simulink model "ctrl_TT"  (R2022b)
settings: Solver=FixedStepAuto  StartTime=0.0  StopTime=Tf  FixedStep=0.05  RelTol=1e-3
InitFcn:
  | run;
StopFcn:
  | save('testdata')
undefined symbols (not defined in the file): Ba_0, Bb, Bv_0, Bx_0, Cp, Cp_prime, d, dA_BP1, dA_BP2, dA_Hull, dA_PH, dA_Sail, dA_SProot, dA_X1a, dA_X1b, dA_X2a, dA_X2b, dA_X3a, dA_X3b, dA_X4a, dA_X4b, Ixx, Ixy, Ixz, Iyy, Iyz, Izz, Mb, n_BP1, n_BP2, n_Hull, n_PH, n_Sail, n_SProot, n_X2a, n_X2b, n_X3a, n_X4a, n_X4b, nt_BP1, nt_BP2, nt_Hull, nt_PH, nt_Sail, nt_SProot, nt_X1a, nt_X1b, nt_X2a, nt_X2b, nt_X3a, nt_X3b, nt_X4a, nt_X4b, Seastate, Tf, vt1_BP1, vt1_BP2, vt1_Hull, vt1_PH, vt1_Sail ... (+44)
libraries: simulink x8, sharedtransform x2, dspmathops x2
(part 4 of 5)

== matlab function ctrl_TT/HDM/HDM B3/Wave, Virtual Mass and Hydrostatic/Wave Particle Motions/Hydrostatic Forces and Moments/Subsystem/MATLAB Function1 ==
  data: time input; Xearth input; Fx_total output; vert1 input; vert2 input; vert3 input; dA input; ntri input; normal input; A_wave input; k_wave input; w_wave input; rho input; g input; Fy_total output; Fz_total output; Mx_total output; My_total output; Mz_total output; Zb input
function [Fx_total,Fy_total,Fz_total,Mx_total,My_total,Mz_total]= fcn(time,Xearth,vert1,vert2,vert3,dA,ntri,normal,A_wave,k_wave,w_wave,rho,g,Zb)
x_e=Xearth(1); y_e=Xearth(2); z_e=Xearth(3);
phi=Xearth(4); theta=Xearth(5); psi=Xearth(6);

RMat=[cos(theta)*cos(psi) -cos(phi)*sin(psi)+sin(phi)*sin(theta)*cos(psi)  sin(phi)*sin(psi)+cos(phi)*sin(theta)*cos(psi); ...
      cos(theta)*sin(psi)  cos(phi)*cos(psi)+sin(phi)*sin(theta)*sin(psi) -sin(phi)*cos(psi)+cos(phi)*sin(theta)*sin(psi); ...
     -sin(theta)                             sin(phi)*cos(theta)                             cos(phi)*cos(theta)];  

%position of mid points in earth coordinate;
mp1=zeros(ntri,3);
mp2=zeros(ntri,3);
mp3=zeros(ntri,3);
nA =zeros(ntri,3);

P1=zeros(ntri,1);
P2=zeros(ntri,1);
P3=zeros(ntri,1);

%position vector of mid points from the CG
r1=zeros(ntri,3);
r2=zeros(ntri,3);
r3=zeros(ntri,3);
v1_w=zeros(ntri,3);
v2_w=zeros(ntri,3);
v3_w=zeros(ntri,3);
n_w=zeros(ntri,3);

%Area of triangle, product of area and unit normal, position vector to each mid-point
for i=1:ntri
    %Area of each triangle
    A=[vert2(i,1)-vert1(i,1); vert2(i,2)-vert1(i,2); vert2(i,3)-vert1(i,3);];
    B=[vert3(i,1)-vert1(i,1); vert3(i,2)-vert1(i,2); vert3(i,3)-vert1(i,3);];
    C=[normal(i,1); normal(i,2); normal(i,3);];
        
    %A*n vector calculation
    for j=1:3
        nA(i,j)=dA(i).*C(j);    
    end
    
    %position vector to each mid point of each edge
    for j=1:3
        r1(i,j)=0.5*(vert1(i,j)+vert2(i,j));
        r2(i,j)=0.5*(vert1(i,j)+vert3(i,j));
        r3(i,j)=0.5*(vert2(i,j)+vert3(i,j));
    end
end

%computing mid point location between vertices in earth coordinate
for i=1:ntri
    MP1=RMat*[r1(i,1); r1(i,2); r1(i,3);]+[x_e; y_e; z_e;];
    MP2=RMat*[r2(i,1); r2(i,2); r2(i,3);]+[x_e; y_e; z_e;];
    MP3=RMat*[r3(i,1); r3(i,2); r3(i,3);]+[x_e; y_e; z_e;];
    
    v1i=RMat*[vert1(i,1); vert1(i,2); vert1(i,3);]+[x_e; y_e; z_e;];
    v2i=RMat*[vert2(i,1); vert2(i,2); vert2(i,3);]+[x_e; y_e; z_e;];
    v3i=RMat*[vert3(i,1); vert3(i,2); vert3(i,3);]+[x_e; y_e; z_e;];
   
    for j=1:3
        v1_w(i,j)=v1i(j); v2_w(i,j)=v2i(j); v3_w(i,j)=v3i(j); 
        mp1(i,j)=MP1(j);  mp2(i,j)=MP2(j);  mp3(i,j)=MP3(j);
    end
end

for i=1:ntri
    A=[v2_w(i,1)-v1_w(i,1); v2_w(i,2)-v1_w(i,2); v2_w(i,3)-v1_w(i,3);];
    B=[v3_w(i,1)-v1_w(i,1); v3_w(i,2)-v1_w(i,2); v3_w(i,3)-v1_w(i,3);];
    n=cross(A,B)/norm(cross(A,B));
    dA(i,1)=0.5*norm(cross(A,B));
    n_w(i,1)=n(1); n_w(i,2)=n(2); n_w(i,3)=n(3);
end


%computing forces and moments for each triangle
Fx_total=0; Fy_total=0; Fz_total=0;
Mx_total=0; My_total=0; Mz_total=0;

for i=1:ntri
    p1=-rho*g*(mp1(i,3)-A_wave*exp(k_wave.*mp1(i,3)).*sin(k_wave*mp1(i,1)-w_wave.*time));
    p2=-rho*g*(mp2(i,3)-A_wave*exp(k_wave.*mp2(i,3)).*sin(k_wave*mp2(i,1)-w_wave.*time));
    p3=-rho*g*(mp3(i,3)-A_wave*exp(k_wave.*mp3(i,3)).*sin(k_wave*mp3(i,1)-w_wave.*time));
    
    dFx=-nA(i,1)*(p1+p2+p3)./3;
    dFy=-nA(i,2)*(p1+p2+p3)./3;
    dFz=-nA(i,3)*(p1+p2+p3)./3;
    
    dP =-p1.*[r1(i,1); r1(i,2); r1(i,3)-Zb;]...
        -p2.*[r2(i,1); r2(i,2); r2(i,3)-Zb;]...
        -p3.*[r3(i,1); r3(i,2); r3(i,3)-Zb;];
    N =[nA(i,1); nA(i,2); nA(i,3);];
    dM=cross(dP,N);
    Fx_total=Fx_total+dFx;
    Fy_total=Fy_total+dFy;
    Fz_total=Fz_total+dFz;
    Mx_total=Mx_total+dM(1)/3;
    My_total=My_total+dM(2)/3;
    Mz_total=Mz_total+dM(3)/3;
end
end

== matlab function ctrl_TT/HDM/HDM B3/Wave, Virtual Mass and Hydrostatic/Wave Particle Motions/Hydrostatic Forces and Moments/Subsystem/MATLAB Function3 ==
  data: time input; Xearth input; Fx_total output; vert1 input; vert2 input; vert3 input; dA input; ntri input; normal input; A_wave input; k_wave input; w_wave input; rho input; g input; Fy_total output; Fz_total output; Mx_total output; My_total output; Mz_total output; Zb input
function [Fx_total,Fy_total,Fz_total,Mx_total,My_total,Mz_total]= fcn(time,Xearth,vert1,vert2,vert3,dA,ntri,normal,A_wave,k_wave,w_wave,rho,g,Zb)
x_e=Xearth(1); y_e=Xearth(2); z_e=Xearth(3);
phi=Xearth(4); theta=Xearth(5); psi=Xearth(6);

RMat=[cos(theta)*cos(psi) -cos(phi)*sin(psi)+sin(phi)*sin(theta)*cos(psi)  sin(phi)*sin(psi)+cos(phi)*sin(theta)*cos(psi); ...
      cos(theta)*sin(psi)  cos(phi)*cos(psi)+sin(phi)*sin(theta)*sin(psi) -sin(phi)*cos(psi)+cos(phi)*sin(theta)*sin(psi); ...
     -sin(theta)                             sin(phi)*cos(theta)                             cos(phi)*cos(theta)];  

%position of mid points in earth coordinate;
mp1=zeros(ntri,3);
mp2=zeros(ntri,3);
mp3=zeros(ntri,3);
nA =zeros(ntri,3);

P1=zeros(ntri,1);
P2=zeros(ntri,1);
P3=zeros(ntri,1);

%position vector of mid points from the CG
r1=zeros(ntri,3);
r2=zeros(ntri,3);
r3=zeros(ntri,3);
v1_w=zeros(ntri,3);
v2_w=zeros(ntri,3);
v3_w=zeros(ntri,3);
n_w=zeros(ntri,3);

%Area of triangle, product of area and unit normal, position vector to each mid-point
for i=1:ntri
    %Area of each triangle
    A=[vert2(i,1)-vert1(i,1); vert2(i,2)-vert1(i,2); vert2(i,3)-vert1(i,3);];
    B=[vert3(i,1)-vert1(i,1); vert3(i,2)-vert1(i,2); vert3(i,3)-vert1(i,3);];
    C=[normal(i,1); normal(i,2); normal(i,3);];
        
    %A*n vector calculation
    for j=1:3
        nA(i,j)=dA(i).*C(j);    
    end
    
    %position vector to each mid point of each edge
    for j=1:3
        r1(i,j)=0.5*(vert1(i,j)+vert2(i,j));
        r2(i,j)=0.5*(vert1(i,j)+vert3(i,j));
        r3(i,j)=0.5*(vert2(i,j)+vert3(i,j));
    end
end

%computing mid point location between vertices in earth coordinate
for i=1:ntri
    MP1=RMat*[r1(i,1); r1(i,2); r1(i,3);]+[x_e; y_e; z_e;];
    MP2=RMat*[r2(i,1); r2(i,2); r2(i,3);]+[x_e; y_e; z_e;];
    MP3=RMat*[r3(i,1); r3(i,2); r3(i,3);]+[x_e; y_e; z_e;];
    
    v1i=RMat*[vert1(i,1); vert1(i,2); vert1(i,3);]+[x_e; y_e; z_e;];
    v2i=RMat*[vert2(i,1); vert2(i,2); vert2(i,3);]+[x_e; y_e; z_e;];
    v3i=RMat*[vert3(i,1); vert3(i,2); vert3(i,3);]+[x_e; y_e; z_e;];
   
    for j=1:3
        v1_w(i,j)=v1i(j); v2_w(i,j)=v2i(j); v3_w(i,j)=v3i(j); 
        mp1(i,j)=MP1(j);  mp2(i,j)=MP2(j);  mp3(i,j)=MP3(j);
    end
end

for i=1:ntri
    A=[v2_w(i,1)-v1_w(i,1); v2_w(i,2)-v1_w(i,2); v2_w(i,3)-v1_w(i,3);];
    B=[v3_w(i,1)-v1_w(i,1); v3_w(i,2)-v1_w(i,2); v3_w(i,3)-v1_w(i,3);];
    n=cross(A,B)/norm(cross(A,B));
    dA(i,1)=0.5*norm(cross(A,B));
    n_w(i,1)=n(1); n_w(i,2)=n(2); n_w(i,3)=n(3);
end



%computing forces and moments for each triangle
Fx_total=0; Fy_total=0; Fz_total=0;
Mx_total=0; My_total=0; Mz_total=0;

for i=1:ntri
    p1=-rho*g*(mp1(i,3)-A_wave*exp(k_wave.*mp1(i,3)).*sin(k_wave*mp1(i,1)-w_wave.*time));
    p2=-rho*g*(mp2(i,3)-A_wave*exp(k_wave.*mp2(i,3)).*sin(k_wave*mp2(i,1)-w_wave.*time));
    p3=-rho*g*(mp3(i,3)-A_wave*exp(k_wave.*mp3(i,3)).*sin(k_wave*mp3(i,1)-w_wave.*time));
    
    dFx=-nA(i,1)*(p1+p2+p3)./3;
    dFy=-nA(i,2)*(p1+p2+p3)./3;
    dFz=-nA(i,3)*(p1+p2+p3)./3;
    
    dP =-p1.*[r1(i,1); r1(i,2); r1(i,3)-Zb;]...
        -p2.*[r2(i,1); r2(i,2); r2(i,3)-Zb;]...
        -p3.*[r3(i,1); r3(i,2); r3(i,3)-Zb;];
    N =[nA(i,1); nA(i,2); nA(i,3);];
    dM=cross(dP,N);
    Fx_total=Fx_total+dFx;
    Fy_total=Fy_total+dFy;
    Fz_total=Fz_total+dFz;
    Mx_total=Mx_total+dM(1)/3;
    My_total=My_total+dM(2)/3;
    Mz_total=Mz_total+dM(3)/3;
end
end

== matlab function ctrl_TT/HDM/HDM B3/Wave, Virtual Mass and Hydrostatic/Wave Particle Motions/Hydrostatic Forces and Moments/Subsystem/MATLAB Function4 ==
  data: time input; Xearth input; Fx_total output; vert1 input; vert2 input; vert3 input; dA input; ntri input; normal input; A_wave input; k_wave input; w_wave input; rho input; g input; Fy_total output; Fz_total output; Mx_total output; My_total output; Mz_total output; Zb input
function [Fx_total,Fy_total,Fz_total,Mx_total,My_total,Mz_total]= fcn(time,Xearth,vert1,vert2,vert3,dA,ntri,normal,A_wave,k_wave,w_wave,rho,g,Zb)
x_e=Xearth(1); y_e=Xearth(2); z_e=Xearth(3);
phi=Xearth(4); theta=Xearth(5); psi=Xearth(6);

RMat=[cos(theta)*cos(psi) -cos(phi)*sin(psi)+sin(phi)*sin(theta)*cos(psi)  sin(phi)*sin(psi)+cos(phi)*sin(theta)*cos(psi); ...
      cos(theta)*sin(psi)  cos(phi)*cos(psi)+sin(phi)*sin(theta)*sin(psi) -sin(phi)*cos(psi)+cos(phi)*sin(theta)*sin(psi); ...
     -sin(theta)                             sin(phi)*cos(theta)                             cos(phi)*cos(theta)];  

%position of mid points in earth coordinate;
mp1=zeros(ntri,3);
mp2=zeros(ntri,3);
mp3=zeros(ntri,3);
nA =zeros(ntri,3);

P1=zeros(ntri,1);
P2=zeros(ntri,1);
P3=zeros(ntri,1);

%position vector of mid points from the CG
r1=zeros(ntri,3);
r2=zeros(ntri,3);
r3=zeros(ntri,3);
v1_w=zeros(ntri,3);
v2_w=zeros(ntri,3);
v3_w=zeros(ntri,3);
n_w=zeros(ntri,3);

%Area of triangle, product of area and unit normal, position vector to each mid-point
for i=1:ntri
    %Area of each triangle
    A=[vert2(i,1)-vert1(i,1); vert2(i,2)-vert1(i,2); vert2(i,3)-vert1(i,3);];
    B=[vert3(i,1)-vert1(i,1); vert3(i,2)-vert1(i,2); vert3(i,3)-vert1(i,3);];
    C=[normal(i,1); normal(i,2); normal(i,3);];
        
    %A*n vector calculation
    for j=1:3
        nA(i,j)=dA(i).*C(j);    
    end
    
    %position vector to each mid point of each edge
    for j=1:3
        r1(i,j)=0.5*(vert1(i,j)+vert2(i,j));
        r2(i,j)=0.5*(vert1(i,j)+vert3(i,j));
        r3(i,j)=0.5*(vert2(i,j)+vert3(i,j));
    end
end

%computing mid point location between vertices in earth coordinate
for i=1:ntri
    MP1=RMat*[r1(i,1); r1(i,2); r1(i,3);]+[x_e; y_e; z_e;];
    MP2=RMat*[r2(i,1); r2(i,2); r2(i,3);]+[x_e; y_e; z_e;];
    MP3=RMat*[r3(i,1); r3(i,2); r3(i,3);]+[x_e; y_e; z_e;];
    
    v1i=RMat*[vert1(i,1); vert1(i,2); vert1(i,3);]+[x_e; y_e; z_e;];
    v2i=RMat*[vert2(i,1); vert2(i,2); vert2(i,3);]+[x_e; y_e; z_e;];
    v3i=RMat*[vert3(i,1); vert3(i,2); vert3(i,3);]+[x_e; y_e; z_e;];
   
    for j=1:3
        v1_w(i,j)=v1i(j); v2_w(i,j)=v2i(j); v3_w(i,j)=v3i(j); 
        mp1(i,j)=MP1(j);  mp2(i,j)=MP2(j);  mp3(i,j)=MP3(j);
    end
end

for i=1:ntri
    A=[v2_w(i,1)-v1_w(i,1); v2_w(i,2)-v1_w(i,2); v2_w(i,3)-v1_w(i,3);];
    B=[v3_w(i,1)-v1_w(i,1); v3_w(i,2)-v1_w(i,2); v3_w(i,3)-v1_w(i,3);];
    n=cross(A,B)/norm(cross(A,B));
    dA(i,1)=0.5*norm(cross(A,B));
    n_w(i,1)=n(1); n_w(i,2)=n(2); n_w(i,3)=n(3);
end


%computing forces and moments for each triangle
Fx_total=0; Fy_total=0; Fz_total=0;
Mx_total=0; My_total=0; Mz_total=0;

for i=1:ntri
    p1=-rho*g*(mp1(i,3)-A_wave*exp(k_wave.*mp1(i,3)).*sin(k_wave*mp1(i,1)-w_wave.*time));
    p2=-rho*g*(mp2(i,3)-A_wave*exp(k_wave.*mp2(i,3)).*sin(k_wave*mp2(i,1)-w_wave.*time));
    p3=-rho*g*(mp3(i,3)-A_wave*exp(k_wave.*mp3(i,3)).*sin(k_wave*mp3(i,1)-w_wave.*time));
    
    dFx=-nA(i,1)*(p1+p2+p3)./3;
    dFy=-nA(i,2)*(p1+p2+p3)./3;
    dFz=-nA(i,3)*(p1+p2+p3)./3;
    
    dP =-p1.*[r1(i,1); r1(i,2); r1(i,3)-Zb;]...
        -p2.*[r2(i,1); r2(i,2); r2(i,3)-Zb;]...
        -p3.*[r3(i,1); r3(i,2); r3(i,3)-Zb;];
    N =[nA(i,1); nA(i,2); nA(i,3);];
    dM=cross(dP,N);
    Fx_total=Fx_total+dFx;
    Fy_total=Fy_total+dFy;
    Fz_total=Fz_total+dFz;
    Mx_total=Mx_total+dM(1)/3;
    My_total=My_total+dM(2)/3;
    Mz_total=Mz_total+dM(3)/3;
end
end

== matlab function ctrl_TT/HDM/HDM B3/Wave, Virtual Mass and Hydrostatic/Wave Particle Motions/Hydrostatic Forces and Moments/Subsystem/MATLAB Function5 ==
  data: time input; Xearth input; Fx_total output; vert1 input; vert2 input; vert3 input; dA input; ntri input; normal input; A_wave input; k_wave input; w_wave input; rho input; g input; Fy_total output; Fz_total output; Mx_total output; My_total output; Mz_total output; Zb input
function [Fx_total,Fy_total,Fz_total,Mx_total,My_total,Mz_total]= fcn(time,Xearth,vert1,vert2,vert3,dA,ntri,normal,A_wave,k_wave,w_wave,rho,g,Zb)
x_e=Xearth(1); y_e=Xearth(2); z_e=Xearth(3);
phi=Xearth(4); theta=Xearth(5); psi=Xearth(6);

RMat=[cos(theta)*cos(psi) -cos(phi)*sin(psi)+sin(phi)*sin(theta)*cos(psi)  sin(phi)*sin(psi)+cos(phi)*sin(theta)*cos(psi); ...
      cos(theta)*sin(psi)  cos(phi)*cos(psi)+sin(phi)*sin(theta)*sin(psi) -sin(phi)*cos(psi)+cos(phi)*sin(theta)*sin(psi); ...
     -sin(theta)                             sin(phi)*cos(theta)                             cos(phi)*cos(theta)];  

%position of mid points in earth coordinate;
mp1=zeros(ntri,3);
mp2=zeros(ntri,3);
mp3=zeros(ntri,3);
nA =zeros(ntri,3);

P1=zeros(ntri,1);
P2=zeros(ntri,1);
P3=zeros(ntri,1);

%position vector of mid points from the CG
r1=zeros(ntri,3);
r2=zeros(ntri,3);
r3=zeros(ntri,3);
v1_w=zeros(ntri,3);
v2_w=zeros(ntri,3);
v3_w=zeros(ntri,3);
n_w=zeros(ntri,3);

%Area of triangle, product of area and unit normal, position vector to each mid-point
for i=1:ntri
    %Area of each triangle
    A=[vert2(i,1)-vert1(i,1); vert2(i,2)-vert1(i,2); vert2(i,3)-vert1(i,3);];
    B=[vert3(i,1)-vert1(i,1); vert3(i,2)-vert1(i,2); vert3(i,3)-vert1(i,3);];
    C=[normal(i,1); normal(i,2); normal(i,3);];
        
    %A*n vector calculation
    for j=1:3
        nA(i,j)=dA(i).*C(j);    
    end
    
    %position vector to each mid point of each edge
    for j=1:3
        r1(i,j)=0.5*(vert1(i,j)+vert2(i,j));
        r2(i,j)=0.5*(vert1(i,j)+vert3(i,j));
        r3(i,j)=0.5*(vert2(i,j)+vert3(i,j));
    end
end

%computing mid point location between vertices in earth coordinate
for i=1:ntri
    MP1=RMat*[r1(i,1); r1(i,2); r1(i,3);]+[x_e; y_e; z_e;];
    MP2=RMat*[r2(i,1); r2(i,2); r2(i,3);]+[x_e; y_e; z_e;];
    MP3=RMat*[r3(i,1); r3(i,2); r3(i,3);]+[x_e; y_e; z_e;];
    
    v1i=RMat*[vert1(i,1); vert1(i,2); vert1(i,3);]+[x_e; y_e; z_e;];
    v2i=RMat*[vert2(i,1); vert2(i,2); vert2(i,3);]+[x_e; y_e; z_e;];
    v3i=RMat*[vert3(i,1); vert3(i,2); vert3(i,3);]+[x_e; y_e; z_e;];
   
    for j=1:3
        v1_w(i,j)=v1i(j); v2_w(i,j)=v2i(j); v3_w(i,j)=v3i(j); 
        mp1(i,j)=MP1(j);  mp2(i,j)=MP2(j);  mp3(i,j)=MP3(j);
    end
end

for i=1:ntri
    A=[v2_w(i,1)-v1_w(i,1); v2_w(i,2)-v1_w(i,2); v2_w(i,3)-v1_w(i,3);];
    B=[v3_w(i,1)-v1_w(i,1); v3_w(i,2)-v1_w(i,2); v3_w(i,3)-v1_w(i,3);];
    n=cross(A,B)/norm(cross(A,B));
    dA(i,1)=0.5*norm(cross(A,B));
    n_w(i,1)=n(1); n_w(i,2)=n(2); n_w(i,3)=n(3);
end



%computing forces and moments for each triangle
Fx_total=0; Fy_total=0; Fz_total=0;
Mx_total=0; My_total=0; Mz_total=0;

for i=1:ntri
    p1=-rho*g*(mp1(i,3)-A_wave*exp(k_wave.*mp1(i,3)).*sin(k_wave*mp1(i,1)-w_wave.*time));
    p2=-rho*g*(mp2(i,3)-A_wave*exp(k_wave.*mp2(i,3)).*sin(k_wave*mp2(i,1)-w_wave.*time));
    p3=-rho*g*(mp3(i,3)-A_wave*exp(k_wave.*mp3(i,3)).*sin(k_wave*mp3(i,1)-w_wave.*time));
    
    dFx=-nA(i,1)*(p1+p2+p3)./3;
    dFy=-nA(i,2)*(p1+p2+p3)./3;
    dFz=-nA(i,3)*(p1+p2+p3)./3;
    
    dP =-p1.*[r1(i,1); r1(i,2); r1(i,3)-Zb;]...
        -p2.*[r2(i,1); r2(i,2); r2(i,3)-Zb;]...
        -p3.*[r3(i,1); r3(i,2); r3(i,3)-Zb;];
    N =[nA(i,1); nA(i,2); nA(i,3);];
    dM=cross(dP,N);
    Fx_total=Fx_total+dFx;
    Fy_total=Fy_total+dFy;
    Fz_total=Fz_total+dFz;
    Mx_total=Mx_total+dM(1)/3;
    My_total=My_total+dM(2)/3;
    Mz_total=Mz_total+dM(3)/3;
end
end

== matlab function ctrl_TT/HDM/HDM B3/Wave, Virtual Mass and Hydrostatic/Wave Particle Motions/Hydrostatic Forces and Moments/X1/MATLAB Function1 ==
  data: time input; Xearth input; Fx_total output; vert1 input; vert2 input; vert3 input; dA input; ntri input; A_wave input; k_wave input; w_wave input; rho input; g input; Fy_total output; Fz_total output; Mx_total output; My_total output; Mz_total output; Zb input; EAX input; dX input; origin input; xcg input
function [Fx_total,Fy_total,Fz_total,Mx_total,My_total,Mz_total]= fcn(time,Xearth,vert1,vert2,vert3,dA,ntri,A_wave,k_wave,w_wave,rho,g,Zb,EAX,dX,origin,xcg)
%EAX=Appendage eulater angle in local coordinate
%its=number of time steps to skip writing grid
x_e=Xearth(1); y_e=Xearth(2); z_e=Xearth(3);
phi=Xearth(4); theta=Xearth(5); psi=Xearth(6);
phiX=EAX(1); thetaX=EAX(2); psiX=EAX(3);


RMat=[cos(theta)*cos(psi) -cos(phi)*sin(psi)+sin(phi)*sin(theta)*cos(psi)  sin(phi)*sin(psi)+cos(phi)*sin(theta)*cos(psi); ...
      cos(theta)*sin(psi)  cos(phi)*cos(psi)+sin(phi)*sin(theta)*sin(psi) -sin(phi)*cos(psi)+cos(phi)*sin(theta)*sin(psi); ...
     -sin(theta)                             sin(phi)*cos(theta)                             cos(phi)*cos(theta)];  
RMATX=[cos(thetaX)*cos(psiX) -cos(phiX)*sin(psiX)+sin(phiX)*sin(thetaX)*cos(psiX)  sin(phiX)*sin(psiX)+cos(phiX)*sin(thetaX)*cos(psiX); ...
      cos(thetaX)*sin(psiX)  cos(phiX)*cos(psiX)+sin(phiX)*sin(thetaX)*sin(psiX) -sin(phiX)*cos(psiX)+cos(phiX)*sin(thetaX)*sin(psiX); ...
     -sin(thetaX)                             sin(phiX)*cos(thetaX)                             cos(phiX)*cos(thetaX)];  
RMATD=[cos(0)*cos(dX) -cos(0)*sin(dX)+sin(0)*sin(0)*cos(dX)  sin(0)*sin(dX)+cos(0)*sin(0)*cos(dX); ...
      cos(0)*sin(dX)  cos(0)*cos(dX)+sin(0)*sin(0)*sin(dX) -sin(0)*cos(dX)+cos(0)*sin(0)*sin(dX); ...
     -sin(0)                             sin(0)*cos(0)                             cos(0)*cos(0)];  


%Rotating the vertices to put in ship coordinate
for i=1:ntri 
    V1=[vert1(i,1); vert1(i,2); vert1(i,3);];
    V2=[vert2(i,1); vert2(i,2); vert2(i,3);];
    V3=[vert3(i,1); vert3(i,2); vert3(i,3);];
        
    %rotating to local z coordinate
    V1_o=inv(RMATX)*(V1-origin*70.2+xcg);
    V2_o=inv(RMATX)*(V2-origin*70.2+xcg);
    V3_o=inv(RMATX)*(V3-origin*70.2+xcg);
    
    %rotating for corresponding appendage deflection
    V1_x=RMATD*V1_o;
    V2_x=RMATD*V2_o;
    V3_x=RMATD*V3_o;
    
        %re-positioning the appendage to local vectors
    V1_r=RMATX*V1_x;
    V2_r=RMATX*V2_x;
    V3_r=RMATX*V3_x;
    
    %re-assigning vertices
    
    for j=1:3
    vert1(i,j)=V1_r(j)+origin(j)*70.2-xcg(j);
    vert2(i,j)=V2_r(j)+origin(j)*70.2-xcg(j);
    vert3(i,j)=V3_r(j)+origin(j)*70.2-xcg(j);
    end  
end

 
%position of mid points in earth coordinate;
mp1=zeros(ntri,3);
mp2=zeros(ntri,3);
mp3=zeros(ntri,3);
nA =zeros(ntri,3);

P1=zeros(ntri,1);
P2=zeros(ntri,1);
P3=zeros(ntri,1);

%position vector of mid points from the CG
r1=zeros(ntri,3);
r2=zeros(ntri,3);
r3=zeros(ntri,3);

v1_w=zeros(ntri,3);
v2_w=zeros(ntri,3);
v3_w=zeros(ntri,3);
n_w=zeros(ntri,3);

%Area of triangle, product of area and unit normal, position vector to each mid-point

for i=1:ntri
    %Area of each triangle
    A=[vert2(i,1)-vert1(i,1); vert2(i,2)-vert1(i,2); vert2(i,3)-vert1(i,3);];
    B=[vert3(i,1)-vert1(i,1); vert3(i,2)-vert1(i,2); vert3(i,3)-vert1(i,3);];
    n=cross(A,B)/norm(cross(A,B));
    C=[n(1); n(2); n(3);];
    %C=[normal(i,1); normal(i,2); normal(i,3);];

    
    %A*n vector calculation
    for j=1:3
        nA(i,j)=dA(i).*C(j);    
    end
    
    %position vector to each mid point of each edge
    for j=1:3
        r1(i,j)=0.5*(vert1(i,j)+vert2(i,j));
        r2(i,j)=0.5*(vert1(i,j)+vert3(i,j));
        r3(i,j)=0.5*(vert2(i,j)+vert3(i,j));
    end
end

%computing mid point location between vertices in earth coordinate
for i=1:ntri
    MP1=RMat*[r1(i,1); r1(i,2); r1(i,3);]+[x_e; y_e; z_e;];
    MP2=RMat*[r2(i,1); r2(i,2); r2(i,3);]+[x_e; y_e; z_e;];
    MP3=RMat*[r3(i,1); r3(i,2); r3(i,3);]+[x_e; y_e; z_e;];
    
    v1i=RMat*[vert1(i,1); vert1(i,2); vert1(i,3);]+[x_e; y_e; z_e;];
    v2i=RMat*[vert2(i,1); vert2(i,2); vert2(i,3);]+[x_e; y_e; z_e;];
    v3i=RMat*[vert3(i,1); vert3(i,2); vert3(i,3);]+[x_e; y_e; z_e;];
    
    for j=1:3
        v1_w(i,j)=v1i(j); v2_w(i,j)=v2i(j); v3_w(i,j)=v3i(j);
        mp1(i,j)=MP1(j);  mp2(i,j)=MP2(j);  mp3(i,j)=MP3(j);
    end
end

for i=1:ntri
    A=[v2_w(i,1)-v1_w(i,1); v2_w(i,2)-v1_w(i,2); v2_w(i,3)-v1_w(i,3);];
    B=[v3_w(i,1)-v1_w(i,1); v3_w(i,2)-v1_w(i,2); v3_w(i,3)-v1_w(i,3);];
    n=cross(A,B)/norm(cross(A,B));
    dA(i,1)=0.5*norm(cross(A,B));
    n_w(i,1)=n(1); n_w(i,2)=n(2); n_w(i,3)=n(3);
end



%computing forces and moments for each triangle
Fx_total=0; Fy_total=0; Fz_total=0;
Mx_total=0; My_total=0; Mz_total=0;

for i=1:ntri
    p1=-rho*g*(mp1(i,3)-A_wave*exp(k_wave.*mp1(i,3)).*sin(k_wave*mp1(i,1)-w_wave.*time));
    p2=-rho*g*(mp2(i,3)-A_wave*exp(k_wave.*mp2(i,3)).*sin(k_wave*mp2(i,1)-w_wave.*time));
    p3=-rho*g*(mp3(i,3)-A_wave*exp(k_wave.*mp3(i,3)).*sin(k_wave*mp3(i,1)-w_wave.*time));
    
    dFx=-nA(i,1)*(p1+p2+p3)./3;
    dFy=-nA(i,2)*(p1+p2+p3)./3;
    dFz=-nA(i,3)*(p1+p2+p3)./3;
    
    dP =-p1.*[r1(i,1); r1(i,2); r1(i,3)-Zb;]...
        -p2.*[r2(i,1); r2(i,2); r2(i,3)-Zb;]...
        -p3.*[r3(i,1); r3(i,2); r3(i,3)-Zb;];
    N =[nA(i,1); nA(i,2); nA(i,3);];
    dM=cross(dP,N);
    Fx_total=Fx_total+dFx;
    Fy_total=Fy_total+dFy;
    Fz_total=Fz_total+dFz;
    Mx_total=Mx_total+dM(1)/3;
    My_total=My_total+dM(2)/3;
    Mz_total=Mz_total+dM(3)/3;
end
end

== matlab function ctrl_TT/HDM/HDM B3/Wave, Virtual Mass and Hydrostatic/Wave Particle Motions/Hydrostatic Forces and Moments/X1/MATLAB Function4 ==
  data: time input; Xearth input; Fx_total output; vert1 input; vert2 input; vert3 input; dA input; ntri input; A_wave input; k_wave input; w_wave input; rho input; g input; Fy_total output; Fz_total output; Mx_total output; My_total output; Mz_total output; Zb input; EAX input; dX input; origin input; xcg input
function [Fx_total,Fy_total,Fz_total,Mx_total,My_total,Mz_total]= fcn(time,Xearth,vert1,vert2,vert3,dA,ntri,A_wave,k_wave,w_wave,rho,g,Zb,EAX,dX,origin,xcg)
%EAX=Appendage eulater angle in local coordinate
%its=number of time steps to skip writing grid

x_e=Xearth(1); y_e=Xearth(2); z_e=Xearth(3);
phi=Xearth(4); theta=Xearth(5); psi=Xearth(6);
phiX=EAX(1); thetaX=EAX(2); psiX=EAX(3);


RMat=[cos(theta)*cos(psi) -cos(phi)*sin(psi)+sin(phi)*sin(theta)*cos(psi)  sin(phi)*sin(psi)+cos(phi)*sin(theta)*cos(psi); ...
      cos(theta)*sin(psi)  cos(phi)*cos(psi)+sin(phi)*sin(theta)*sin(psi) -sin(phi)*cos(psi)+cos(phi)*sin(theta)*sin(psi); ...
     -sin(theta)                             sin(phi)*cos(theta)                             cos(phi)*cos(theta)];  
RMATX=[cos(thetaX)*cos(psiX) -cos(phiX)*sin(psiX)+sin(phiX)*sin(thetaX)*cos(psiX)  sin(phiX)*sin(psiX)+cos(phiX)*sin(thetaX)*cos(psiX); ...
      cos(thetaX)*sin(psiX)  cos(phiX)*cos(psiX)+sin(phiX)*sin(thetaX)*sin(psiX) -sin(phiX)*cos(psiX)+cos(phiX)*sin(thetaX)*sin(psiX); ...
     -sin(thetaX)                             sin(phiX)*cos(thetaX)                             cos(phiX)*cos(thetaX)];  
RMATD=[cos(0)*cos(dX) -cos(0)*sin(dX)+sin(0)*sin(0)*cos(dX)  sin(0)*sin(dX)+cos(0)*sin(0)*cos(dX); ...
      cos(0)*sin(dX)  cos(0)*cos(dX)+sin(0)*sin(0)*sin(dX) -sin(0)*cos(dX)+cos(0)*sin(0)*sin(dX); ...
     -sin(0)                             sin(0)*cos(0)                             cos(0)*cos(0)];  


%Rotating the vertices to put in ship coordinate
for i=1:ntri 
    V1=[vert1(i,1); vert1(i,2); vert1(i,3);];
    V2=[vert2(i,1); vert2(i,2); vert2(i,3);];
    V3=[vert3(i,1); vert3(i,2); vert3(i,3);];
        
    %rotating to local z coordinate
    V1_o=inv(RMATX)*(V1-origin*70.2+xcg);
    V2_o=inv(RMATX)*(V2-origin*70.2+xcg);
    V3_o=inv(RMATX)*(V3-origin*70.2+xcg);
    
    %rotating for corresponding appendage deflection
    V1_x=RMATD*V1_o;
    V2_x=RMATD*V2_o;
    V3_x=RMATD*V3_o;
    
        %re-positioning the appendage to local vectors
    V1_r=RMATX*V1_x;
    V2_r=RMATX*V2_x;
    V3_r=RMATX*V3_x;
    
    %re-assigning vertices
    
    for j=1:3
    vert1(i,j)=V1_r(j)+origin(j)*70.2-xcg(j);
    vert2(i,j)=V2_r(j)+origin(j)*70.2-xcg(j);
    vert3(i,j)=V3_r(j)+origin(j)*70.2-xcg(j);
    end  
end

 
%position of mid points in earth coordinate;
mp1=zeros(ntri,3);
mp2=zeros(ntri,3);
mp3=zeros(ntri,3);
nA =zeros(ntri,3);

P1=zeros(ntri,1);
P2=zeros(ntri,1);
P3=zeros(ntri,1);

%position vector of mid points from the CG
r1=zeros(ntri,3);
r2=zeros(ntri,3);
r3=zeros(ntri,3);

v1_w=zeros(ntri,3);
v2_w=zeros(ntri,3);
v3_w=zeros(ntri,3);
n_w=zeros(ntri,3);

%Area of triangle, product of area and unit normal, position vector to each mid-point

for i=1:ntri
    %Area of each triangle
    A=[vert2(i,1)-vert1(i,1); vert2(i,2)-vert1(i,2); vert2(i,3)-vert1(i,3);];
    B=[vert3(i,1)-vert1(i,1); vert3(i,2)-vert1(i,2); vert3(i,3)-vert1(i,3);];
    n=cross(A,B)/norm(cross(A,B));
    C=[n(1); n(2); n(3);];
    %C=[normal(i,1); normal(i,2); normal(i,3);];

    
    %A*n vector calculation
    for j=1:3
        nA(i,j)=dA(i).*C(j);    
    end
    
    %position vector to each mid point of each edge
    for j=1:3
        r1(i,j)=0.5*(vert1(i,j)+vert2(i,j));
        r2(i,j)=0.5*(vert1(i,j)+vert3(i,j));
        r3(i,j)=0.5*(vert2(i,j)+vert3(i,j));
    end
end

%computing mid point location between vertices in earth coordinate
for i=1:ntri
    MP1=RMat*[r1(i,1); r1(i,2); r1(i,3);]+[x_e; y_e; z_e;];
    MP2=RMat*[r2(i,1); r2(i,2); r2(i,3);]+[x_e; y_e; z_e;];
    MP3=RMat*[r3(i,1); r3(i,2); r3(i,3);]+[x_e; y_e; z_e;];
    
    v1i=RMat*[vert1(i,1); vert1(i,2); vert1(i,3);]+[x_e; y_e; z_e;];
    v2i=RMat*[vert2(i,1); vert2(i,2); vert2(i,3);]+[x_e; y_e; z_e;];
    v3i=RMat*[vert3(i,1); vert3(i,2); vert3(i,3);]+[x_e; y_e; z_e;];
    
    for j=1:3
        v1_w(i,j)=v1i(j); v2_w(i,j)=v2i(j); v3_w(i,j)=v3i(j);
        mp1(i,j)=MP1(j);  mp2(i,j)=MP2(j);  mp3(i,j)=MP3(j);
    end
end

for i=1:ntri
    A=[v2_w(i,1)-v1_w(i,1); v2_w(i,2)-v1_w(i,2); v2_w(i,3)-v1_w(i,3);];
    B=[v3_w(i,1)-v1_w(i,1); v3_w(i,2)-v1_w(i,2); v3_w(i,3)-v1_w(i,3);];
    n=cross(A,B)/norm(cross(A,B));
    dA(i,1)=0.5*norm(cross(A,B));
    n_w(i,1)=n(1); n_w(i,2)=n(2); n_w(i,3)=n(3);
end



%computing forces and moments for each triangle
Fx_total=0; Fy_total=0; Fz_total=0;
Mx_total=0; My_total=0; Mz_total=0;

for i=1:ntri
    p1=-rho*g*(mp1(i,3)-A_wave*exp(k_wave.*mp1(i,3)).*sin(k_wave*mp1(i,1)-w_wave.*time));
    p2=-rho*g*(mp2(i,3)-A_wave*exp(k_wave.*mp2(i,3)).*sin(k_wave*mp2(i,1)-w_wave.*time));
    p3=-rho*g*(mp3(i,3)-A_wave*exp(k_wave.*mp3(i,3)).*sin(k_wave*mp3(i,1)-w_wave.*time));
    
    dFx=-nA(i,1)*(p1+p2+p3)./3;
    dFy=-nA(i,2)*(p1+p2+p3)./3;
    dFz=-nA(i,3)*(p1+p2+p3)./3;
    
    dP =-p1.*[r1(i,1); r1(i,2); r1(i,3)-Zb;]...
        -p2.*[r2(i,1); r2(i,2); r2(i,3)-Zb;]...
        -p3.*[r3(i,1); r3(i,2); r3(i,3)-Zb;];
    N =[nA(i,1); nA(i,2); nA(i,3);];
    dM=cross(dP,N);
    Fx_total=Fx_total+dFx;
    Fy_total=Fy_total+dFy;
    Fz_total=Fz_total+dFz;
    Mx_total=Mx_total+dM(1)/3;
    My_total=My_total+dM(2)/3;
    Mz_total=Mz_total+dM(3)/3;
end
end

== matlab function ctrl_TT/HDM/HDM B3/Wave, Virtual Mass and Hydrostatic/Wave Particle Motions/Hydrostatic Forces and Moments/X2/MATLAB Function1 ==
  data: time input; Xearth input; Fx_total output; vert1 input; vert2 input; vert3 input; dA input; ntri input; A_wave input; k_wave input; w_wave input; rho input; g input; Fy_total output; Fz_total output; Mx_total output; My_total output; Mz_total output; Zb input; EAX input; dX input; origin input; xcg input
function [Fx_total,Fy_total,Fz_total,Mx_total,My_total,Mz_total]= fcn(time,Xearth,vert1,vert2,vert3,dA,ntri,A_wave,k_wave,w_wave,rho,g,Zb,EAX,dX,origin,xcg)
%EAX=Appendage eulater angle in local coordinate
%its=number of time steps to skip writing grid

x_e=Xearth(1); y_e=Xearth(2); z_e=Xearth(3);
phi=Xearth(4); theta=Xearth(5); psi=Xearth(6);
phiX=EAX(1); thetaX=EAX(2); psiX=EAX(3);


RMat=[cos(theta)*cos(psi) -cos(phi)*sin(psi)+sin(phi)*sin(theta)*cos(psi)  sin(phi)*sin(psi)+cos(phi)*sin(theta)*cos(psi); ...
      cos(theta)*sin(psi)  cos(phi)*cos(psi)+sin(phi)*sin(theta)*sin(psi) -sin(phi)*cos(psi)+cos(phi)*sin(theta)*sin(psi); ...
     -sin(theta)                             sin(phi)*cos(theta)                             cos(phi)*cos(theta)];  
RMATX=[cos(thetaX)*cos(psiX) -cos(phiX)*sin(psiX)+sin(phiX)*sin(thetaX)*cos(psiX)  sin(phiX)*sin(psiX)+cos(phiX)*sin(thetaX)*cos(psiX); ...
      cos(thetaX)*sin(psiX)  cos(phiX)*cos(psiX)+sin(phiX)*sin(thetaX)*sin(psiX) -sin(phiX)*cos(psiX)+cos(phiX)*sin(thetaX)*sin(psiX); ...
     -sin(thetaX)                             sin(phiX)*cos(thetaX)                             cos(phiX)*cos(thetaX)];  
RMATD=[cos(0)*cos(dX) -cos(0)*sin(dX)+sin(0)*sin(0)*cos(dX)  sin(0)*sin(dX)+cos(0)*sin(0)*cos(dX); ...
      cos(0)*sin(dX)  cos(0)*cos(dX)+sin(0)*sin(0)*sin(dX) -sin(0)*cos(dX)+cos(0)*sin(0)*sin(dX); ...
     -sin(0)                             sin(0)*cos(0)                             cos(0)*cos(0)];  


%Rotating the vertices to put in ship coordinate
for i=1:ntri 
    V1=[vert1(i,1); vert1(i,2); vert1(i,3);];
    V2=[vert2(i,1); vert2(i,2); vert2(i,3);];
    V3=[vert3(i,1); vert3(i,2); vert3(i,3);];
        
    %rotating to local z coordinate
    V1_o=inv(RMATX)*(V1-origin*70.2+xcg);
    V2_o=inv(RMATX)*(V2-origin*70.2+xcg);
    V3_o=inv(RMATX)*(V3-origin*70.2+xcg);
    
    %rotating for corresponding appendage deflection
    V1_x=RMATD*V1_o;
    V2_x=RMATD*V2_o;
    V3_x=RMATD*V3_o;
    
        %re-positioning the appendage to local vectors
    V1_r=RMATX*V1_x;
    V2_r=RMATX*V2_x;
    V3_r=RMATX*V3_x;
    
    %re-assigning vertices
    
    for j=1:3
    vert1(i,j)=V1_r(j)+origin(j)*70.2-xcg(j);
    vert2(i,j)=V2_r(j)+origin(j)*70.2-xcg(j);
    vert3(i,j)=V3_r(j)+origin(j)*70.2-xcg(j);
    end  
end

 
%position of mid points in earth coordinate;
mp1=zeros(ntri,3);
mp2=zeros(ntri,3);
mp3=zeros(ntri,3);
nA =zeros(ntri,3);

P1=zeros(ntri,1);
P2=zeros(ntri,1);
P3=zeros(ntri,1);

%position vector of mid points from the CG
r1=zeros(ntri,3);
r2=zeros(ntri,3);
r3=zeros(ntri,3);

v1_w=zeros(ntri,3);
v2_w=zeros(ntri,3);
v3_w=zeros(ntri,3);
n_w=zeros(ntri,3);

%Area of triangle, product of area and unit normal, position vector to each mid-point

for i=1:ntri
    %Area of each triangle
    A=[vert2(i,1)-vert1(i,1); vert2(i,2)-vert1(i,2); vert2(i,3)-vert1(i,3);];
    B=[vert3(i,1)-vert1(i,1); vert3(i,2)-vert1(i,2); vert3(i,3)-vert1(i,3);];
    n=cross(A,B)/norm(cross(A,B));
    C=[n(1); n(2); n(3);];
    %C=[normal(i,1); normal(i,2); normal(i,3);];

    
    %A*n vector calculation
    for j=1:3
        nA(i,j)=dA(i).*C(j);    
    end
    
    %position vector to each mid point of each edge
    for j=1:3
        r1(i,j)=0.5*(vert1(i,j)+vert2(i,j));
        r2(i,j)=0.5*(vert1(i,j)+vert3(i,j));
        r3(i,j)=0.5*(vert2(i,j)+vert3(i,j));
    end
end

%computing mid point location between vertices in earth coordinate
for i=1:ntri
    MP1=RMat*[r1(i,1); r1(i,2); r1(i,3);]+[x_e; y_e; z_e;];
    MP2=RMat*[r2(i,1); r2(i,2); r2(i,3);]+[x_e; y_e; z_e;];
    MP3=RMat*[r3(i,1); r3(i,2); r3(i,3);]+[x_e; y_e; z_e;];
    
    v1i=RMat*[vert1(i,1); vert1(i,2); vert1(i,3);]+[x_e; y_e; z_e;];
    v2i=RMat*[vert2(i,1); vert2(i,2); vert2(i,3);]+[x_e; y_e; z_e;];
    v3i=RMat*[vert3(i,1); vert3(i,2); vert3(i,3);]+[x_e; y_e; z_e;];
    
    for j=1:3
        v1_w(i,j)=v1i(j); v2_w(i,j)=v2i(j); v3_w(i,j)=v3i(j);
        mp1(i,j)=MP1(j);  mp2(i,j)=MP2(j);  mp3(i,j)=MP3(j);
    end
end

for i=1:ntri
    A=[v2_w(i,1)-v1_w(i,1); v2_w(i,2)-v1_w(i,2); v2_w(i,3)-v1_w(i,3);];
    B=[v3_w(i,1)-v1_w(i,1); v3_w(i,2)-v1_w(i,2); v3_w(i,3)-v1_w(i,3);];
    n=cross(A,B)/norm(cross(A,B));
    dA(i,1)=0.5*norm(cross(A,B));
    n_w(i,1)=n(1); n_w(i,2)=n(2); n_w(i,3)=n(3);
end


%computing forces and moments for each triangle
Fx_total=0; Fy_total=0; Fz_total=0;
Mx_total=0; My_total=0; Mz_total=0;

for i=1:ntri
    p1=-rho*g*(mp1(i,3)-A_wave*exp(k_wave.*mp1(i,3)).*sin(k_wave*mp1(i,1)-w_wave.*time));
    p2=-rho*g*(mp2(i,3)-A_wave*exp(k_wave.*mp2(i,3)).*sin(k_wave*mp2(i,1)-w_wave.*time));
    p3=-rho*g*(mp3(i,3)-A_wave*exp(k_wave.*mp3(i,3)).*sin(k_wave*mp3(i,1)-w_wave.*time));
    
    dFx=-nA(i,1)*(p1+p2+p3)./3;
    dFy=-nA(i,2)*(p1+p2+p3)./3;
    dFz=-nA(i,3)*(p1+p2+p3)./3;
    
    dP =-p1.*[r1(i,1); r1(i,2); r1(i,3)-Zb;]...
        -p2.*[r2(i,1); r2(i,2); r2(i,3)-Zb;]...
        -p3.*[r3(i,1); r3(i,2); r3(i,3)-Zb;];
    N =[nA(i,1); nA(i,2); nA(i,3);];
    dM=cross(dP,N);
    Fx_total=Fx_total+dFx;
    Fy_total=Fy_total+dFy;
    Fz_total=Fz_total+dFz;
    Mx_total=Mx_total+dM(1)/3;
    My_total=My_total+dM(2)/3;
    Mz_total=Mz_total+dM(3)/3;
end
end

== matlab function ctrl_TT/HDM/HDM B3/Wave, Virtual Mass and Hydrostatic/Wave Particle Motions/Hydrostatic Forces and Moments/X2/MATLAB Function4 ==
  data: time input; Xearth input; Fx_total output; vert1 input; vert2 input; vert3 input; dA input; ntri input; A_wave input; k_wave input; w_wave input; rho input; g input; Fy_total output; Fz_total output; Mx_total output; My_total output; Mz_total output; Zb input; EAX input; dX input; origin input; xcg input
function [Fx_total,Fy_total,Fz_total,Mx_total,My_total,Mz_total]= fcn(time,Xearth,vert1,vert2,vert3,dA,ntri,A_wave,k_wave,w_wave,rho,g,Zb,EAX,dX,origin,xcg)
%EAX=Appendage eulater angle in local coordinate
%its=number of time steps to skip writing grid

x_e=Xearth(1); y_e=Xearth(2); z_e=Xearth(3);
phi=Xearth(4); theta=Xearth(5); psi=Xearth(6);
phiX=EAX(1); thetaX=EAX(2); psiX=EAX(3);


RMat=[cos(theta)*cos(psi) -cos(phi)*sin(psi)+sin(phi)*sin(theta)*cos(psi)  sin(phi)*sin(psi)+cos(phi)*sin(theta)*cos(psi); ...
      cos(theta)*sin(psi)  cos(phi)*cos(psi)+sin(phi)*sin(theta)*sin(psi) -sin(phi)*cos(psi)+cos(phi)*sin(theta)*sin(psi); ...
     -sin(theta)                             sin(phi)*cos(theta)                             cos(phi)*cos(theta)];  
RMATX=[cos(thetaX)*cos(psiX) -cos(phiX)*sin(psiX)+sin(phiX)*sin(thetaX)*cos(psiX)  sin(phiX)*sin(psiX)+cos(phiX)*sin(thetaX)*cos(psiX); ...
      cos(thetaX)*sin(psiX)  cos(phiX)*cos(psiX)+sin(phiX)*sin(thetaX)*sin(psiX) -sin(phiX)*cos(psiX)+cos(phiX)*sin(thetaX)*sin(psiX); ...
     -sin(thetaX)                             sin(phiX)*cos(thetaX)                             cos(phiX)*cos(thetaX)];  
RMATD=[cos(0)*cos(dX) -cos(0)*sin(dX)+sin(0)*sin(0)*cos(dX)  sin(0)*sin(dX)+cos(0)*sin(0)*cos(dX); ...
      cos(0)*sin(dX)  cos(0)*cos(dX)+sin(0)*sin(0)*sin(dX) -sin(0)*cos(dX)+cos(0)*sin(0)*sin(dX); ...
     -sin(0)                             sin(0)*cos(0)                             cos(0)*cos(0)];  


%Rotating the vertices to put in ship coordinate
for i=1:ntri 
    V1=[vert1(i,1); vert1(i,2); vert1(i,3);];
    V2=[vert2(i,1); vert2(i,2); vert2(i,3);];
    V3=[vert3(i,1); vert3(i,2); vert3(i,3);];
        
    %rotating to local z coordinate
    V1_o=inv(RMATX)*(V1-origin*70.2+xcg);
    V2_o=inv(RMATX)*(V2-origin*70.2+xcg);
    V3_o=inv(RMATX)*(V3-origin*70.2+xcg);
    
    %rotating for corresponding appendage deflection
    V1_x=RMATD*V1_o;
    V2_x=RMATD*V2_o;
    V3_x=RMATD*V3_o;
    
        %re-positioning the appendage to local vectors
    V1_r=RMATX*V1_x;
    V2_r=RMATX*V2_x;
    V3_r=RMATX*V3_x;
    
    %re-assigning vertices
    
    for j=1:3
    vert1(i,j)=V1_r(j)+origin(j)*70.2-xcg(j);
    vert2(i,j)=V2_r(j)+origin(j)*70.2-xcg(j);
    vert3(i,j)=V3_r(j)+origin(j)*70.2-xcg(j);
    end  
end

 
%position of mid points in earth coordinate;
mp1=zeros(ntri,3);
mp2=zeros(ntri,3);
mp3=zeros(ntri,3);
nA =zeros(ntri,3);

P1=zeros(ntri,1);
P2=zeros(ntri,1);
P3=zeros(ntri,1);

%position vector of mid points from the CG
r1=zeros(ntri,3);
r2=zeros(ntri,3);
r3=zeros(ntri,3);

v1_w=zeros(ntri,3);
v2_w=zeros(ntri,3);
v3_w=zeros(ntri,3);
n_w=zeros(ntri,3);

%Area of triangle, product of area and unit normal, position vector to each mid-point

for i=1:ntri
    %Area of each triangle
    A=[vert2(i,1)-vert1(i,1); vert2(i,2)-vert1(i,2); vert2(i,3)-vert1(i,3);];
    B=[vert3(i,1)-vert1(i,1); vert3(i,2)-vert1(i,2); vert3(i,3)-vert1(i,3);];
    n=cross(A,B)/norm(cross(A,B));
    C=[n(1); n(2); n(3);];
    %C=[normal(i,1); normal(i,2); normal(i,3);];

    
    %A*n vector calculation
    for j=1:3
        nA(i,j)=dA(i).*C(j);    
    end
    
    %position vector to each mid point of each edge
    for j=1:3
        r1(i,j)=0.5*(vert1(i,j)+vert2(i,j));
        r2(i,j)=0.5*(vert1(i,j)+vert3(i,j));
        r3(i,j)=0.5*(vert2(i,j)+vert3(i,j));
    end
end

%computing mid point location between vertices in earth coordinate
for i=1:ntri
    MP1=RMat*[r1(i,1); r1(i,2); r1(i,3);]+[x_e; y_e; z_e;];
    MP2=RMat*[r2(i,1); r2(i,2); r2(i,3);]+[x_e; y_e; z_e;];
    MP3=RMat*[r3(i,1); r3(i,2); r3(i,3);]+[x_e; y_e; z_e;];
    
    v1i=RMat*[vert1(i,1); vert1(i,2); vert1(i,3);]+[x_e; y_e; z_e;];
    v2i=RMat*[vert2(i,1); vert2(i,2); vert2(i,3);]+[x_e; y_e; z_e;];
    v3i=RMat*[vert3(i,1); vert3(i,2); vert3(i,3);]+[x_e; y_e; z_e;];
    
    for j=1:3
        v1_w(i,j)=v1i(j); v2_w(i,j)=v2i(j); v3_w(i,j)=v3i(j);
        mp1(i,j)=MP1(j);  mp2(i,j)=MP2(j);  mp3(i,j)=MP3(j);
    end
end

for i=1:ntri
    A=[v2_w(i,1)-v1_w(i,1); v2_w(i,2)-v1_w(i,2); v2_w(i,3)-v1_w(i,3);];
    B=[v3_w(i,1)-v1_w(i,1); v3_w(i,2)-v1_w(i,2); v3_w(i,3)-v1_w(i,3);];
    n=cross(A,B)/norm(cross(A,B));
    dA(i,1)=0.5*norm(cross(A,B));
    n_w(i,1)=n(1); n_w(i,2)=n(2); n_w(i,3)=n(3);
end



%computing forces and moments for each triangle
Fx_total=0; Fy_total=0; Fz_total=0;
Mx_total=0; My_total=0; Mz_total=0;

for i=1:ntri
    p1=-rho*g*(mp1(i,3)-A_wave*exp(k_wave.*mp1(i,3)).*sin(k_wave*mp1(i,1)-w_wave.*time));
    p2=-rho*g*(mp2(i,3)-A_wave*exp(k_wave.*mp2(i,3)).*sin(k_wave*mp2(i,1)-w_wave.*time));
    p3=-rho*g*(mp3(i,3)-A_wave*exp(k_wave.*mp3(i,3)).*sin(k_wave*mp3(i,1)-w_wave.*time));
    
    dFx=-nA(i,1)*(p1+p2+p3)./3;
    dFy=-nA(i,2)*(p1+p2+p3)./3;
    dFz=-nA(i,3)*(p1+p2+p3)./3;
    
    dP =-p1.*[r1(i,1); r1(i,2); r1(i,3)-Zb;]...
        -p2.*[r2(i,1); r2(i,2); r2(i,3)-Zb;]...
        -p3.*[r3(i,1); r3(i,2); r3(i,3)-Zb;];
    N =[nA(i,1); nA(i,2); nA(i,3);];
    dM=cross(dP,N);
    Fx_total=Fx_total+dFx;
    Fy_total=Fy_total+dFy;
    Fz_total=Fz_total+dFz;
    Mx_total=Mx_total+dM(1)/3;
    My_total=My_total+dM(2)/3;
    Mz_total=Mz_total+dM(3)/3;
end
end

== matlab function ctrl_TT/HDM/HDM B3/Wave, Virtual Mass and Hydrostatic/Wave Particle Motions/Hydrostatic Forces and Moments/X3/MATLAB Function1 ==
  data: time input; Xearth input; Fx_total output; vert1 input; vert2 input; vert3 input; dA input; ntri input; A_wave input; k_wave input; w_wave input; rho input; g input; Fy_total output; Fz_total output; Mx_total output; My_total output; Mz_total output; Zb input; EAX input; dX input; origin input; xcg input
function [Fx_total,Fy_total,Fz_total,Mx_total,My_total,Mz_total]= fcn(time,Xearth,vert1,vert2,vert3,dA,ntri,A_wave,k_wave,w_wave,rho,g,Zb,EAX,dX,origin,xcg)
%EAX=Appendage eulater angle in local coordinate
%its=number of time steps to skip writing grid

x_e=Xearth(1); y_e=Xearth(2); z_e=Xearth(3);
phi=Xearth(4); theta=Xearth(5); psi=Xearth(6);
phiX=EAX(1); thetaX=EAX(2); psiX=EAX(3);


RMat=[cos(theta)*cos(psi) -cos(phi)*sin(psi)+sin(phi)*sin(theta)*cos(psi)  sin(phi)*sin(psi)+cos(phi)*sin(theta)*cos(psi); ...
      cos(theta)*sin(psi)  cos(phi)*cos(psi)+sin(phi)*sin(theta)*sin(psi) -sin(phi)*cos(psi)+cos(phi)*sin(theta)*sin(psi); ...
     -sin(theta)                             sin(phi)*cos(theta)                             cos(phi)*cos(theta)];  
RMATX=[cos(thetaX)*cos(psiX) -cos(phiX)*sin(psiX)+sin(phiX)*sin(thetaX)*cos(psiX)  sin(phiX)*sin(psiX)+cos(phiX)*sin(thetaX)*cos(psiX); ...
      cos(thetaX)*sin(psiX)  cos(phiX)*cos(psiX)+sin(phiX)*sin(thetaX)*sin(psiX) -sin(phiX)*cos(psiX)+cos(phiX)*sin(thetaX)*sin(psiX); ...
     -sin(thetaX)                             sin(phiX)*cos(thetaX)                             cos(phiX)*cos(thetaX)];  
RMATD=[cos(0)*cos(dX) -cos(0)*sin(dX)+sin(0)*sin(0)*cos(dX)  sin(0)*sin(dX)+cos(0)*sin(0)*cos(dX); ...
      cos(0)*sin(dX)  cos(0)*cos(dX)+sin(0)*sin(0)*sin(dX) -sin(0)*cos(dX)+cos(0)*sin(0)*sin(dX); ...
     -sin(0)                             sin(0)*cos(0)                             cos(0)*cos(0)];  


%Rotating the vertices to put in ship coordinate
for i=1:ntri 
    V1=[vert1(i,1); vert1(i,2); vert1(i,3);];
    V2=[vert2(i,1); vert2(i,2); vert2(i,3);];
    V3=[vert3(i,1); vert3(i,2); vert3(i,3);];
        
    %rotating to local z coordinate
    V1_o=inv(RMATX)*(V1-origin*70.2+xcg);
    V2_o=inv(RMATX)*(V2-origin*70.2+xcg);
    V3_o=inv(RMATX)*(V3-origin*70.2+xcg);
    
    %rotating for corresponding appendage deflection
    V1_x=RMATD*V1_o;
    V2_x=RMATD*V2_o;
    V3_x=RMATD*V3_o;
    
        %re-positioning the appendage to local vectors
    V1_r=RMATX*V1_x;
    V2_r=RMATX*V2_x;
    V3_r=RMATX*V3_x;
    
    %re-assigning vertices
    
    for j=1:3
    vert1(i,j)=V1_r(j)+origin(j)*70.2-xcg(j);
    vert2(i,j)=V2_r(j)+origin(j)*70.2-xcg(j);
    vert3(i,j)=V3_r(j)+origin(j)*70.2-xcg(j);
    end  
end

 
%position of mid points in earth coordinate;
mp1=zeros(ntri,3);
mp2=zeros(ntri,3);
mp3=zeros(ntri,3);
nA =zeros(ntri,3);

P1=zeros(ntri,1);
P2=zeros(ntri,1);
P3=zeros(ntri,1);

%position vector of mid points from the CG
r1=zeros(ntri,3);
r2=zeros(ntri,3);
r3=zeros(ntri,3);

v1_w=zeros(ntri,3);
v2_w=zeros(ntri,3);
v3_w=zeros(ntri,3);
n_w=zeros(ntri,3);

%Area of triangle, product of area and unit normal, position vector to each mid-point

for i=1:ntri
    %Area of each triangle
    A=[vert2(i,1)-vert1(i,1); vert2(i,2)-vert1(i,2); vert2(i,3)-vert1(i,3);];
    B=[vert3(i,1)-vert1(i,1); vert3(i,2)-vert1(i,2); vert3(i,3)-vert1(i,3);];
    n=cross(A,B)/norm(cross(A,B));
    C=[n(1); n(2); n(3);];
    %C=[normal(i,1); normal(i,2); normal(i,3);];

    
    %A*n vector calculation
    for j=1:3
        nA(i,j)=dA(i).*C(j);    
    end
    
    %position vector to each mid point of each edge
    for j=1:3
        r1(i,j)=0.5*(vert1(i,j)+vert2(i,j));
        r2(i,j)=0.5*(vert1(i,j)+vert3(i,j));
        r3(i,j)=0.5*(vert2(i,j)+vert3(i,j));
    end
end

%computing mid point location between vertices in earth coordinate
for i=1:ntri
    MP1=RMat*[r1(i,1); r1(i,2); r1(i,3);]+[x_e; y_e; z_e;];
    MP2=RMat*[r2(i,1); r2(i,2); r2(i,3);]+[x_e; y_e; z_e;];
    MP3=RMat*[r3(i,1); r3(i,2); r3(i,3);]+[x_e; y_e; z_e;];
    
    v1i=RMat*[vert1(i,1); vert1(i,2); vert1(i,3);]+[x_e; y_e; z_e;];
    v2i=RMat*[vert2(i,1); vert2(i,2); vert2(i,3);]+[x_e; y_e; z_e;];
    v3i=RMat*[vert3(i,1); vert3(i,2); vert3(i,3);]+[x_e; y_e; z_e;];
    
    for j=1:3
        v1_w(i,j)=v1i(j); v2_w(i,j)=v2i(j); v3_w(i,j)=v3i(j);
        mp1(i,j)=MP1(j);  mp2(i,j)=MP2(j);  mp3(i,j)=MP3(j);
    end
end

for i=1:ntri
    A=[v2_w(i,1)-v1_w(i,1); v2_w(i,2)-v1_w(i,2); v2_w(i,3)-v1_w(i,3);];
    B=[v3_w(i,1)-v1_w(i,1); v3_w(i,2)-v1_w(i,2); v3_w(i,3)-v1_w(i,3);];
    n=cross(A,B)/norm(cross(A,B));
    dA(i,1)=0.5*norm(cross(A,B));
    n_w(i,1)=n(1); n_w(i,2)=n(2); n_w(i,3)=n(3);
end



%computing forces and moments for each triangle
Fx_total=0; Fy_total=0; Fz_total=0;
Mx_total=0; My_total=0; Mz_total=0;

for i=1:ntri
    p1=-rho*g*(mp1(i,3)-A_wave*exp(k_wave.*mp1(i,3)).*sin(k_wave*mp1(i,1)-w_wave.*time));
    p2=-rho*g*(mp2(i,3)-A_wave*exp(k_wave.*mp2(i,3)).*sin(k_wave*mp2(i,1)-w_wave.*time));
    p3=-rho*g*(mp3(i,3)-A_wave*exp(k_wave.*mp3(i,3)).*sin(k_wave*mp3(i,1)-w_wave.*time));
    
    dFx=-nA(i,1)*(p1+p2+p3)./3;
    dFy=-nA(i,2)*(p1+p2+p3)./3;
    dFz=-nA(i,3)*(p1+p2+p3)./3;
    
    dP =-p1.*[r1(i,1); r1(i,2); r1(i,3)-Zb;]...
        -p2.*[r2(i,1); r2(i,2); r2(i,3)-Zb;]...
        -p3.*[r3(i,1); r3(i,2); r3(i,3)-Zb;];
    N =[nA(i,1); nA(i,2); nA(i,3);];
    dM=cross(dP,N);
    Fx_total=Fx_total+dFx;
    Fy_total=Fy_total+dFy;
    Fz_total=Fz_total+dFz;
    Mx_total=Mx_total+dM(1)/3;
    My_total=My_total+dM(2)/3;
    Mz_total=Mz_total+dM(3)/3;
end
end

== matlab function ctrl_TT/HDM/HDM B3/Wave, Virtual Mass and Hydrostatic/Wave Particle Motions/Hydrostatic Forces and Moments/X3/MATLAB Function4 ==
  data: time input; Xearth input; Fx_total output; vert1 input; vert2 input; vert3 input; dA input; ntri input; A_wave input; k_wave input; w_wave input; rho input; g input; Fy_total output; Fz_total output; Mx_total output; My_total output; Mz_total output; Zb input; EAX input; dX input; origin input; xcg input
function [Fx_total,Fy_total,Fz_total,Mx_total,My_total,Mz_total]= fcn(time,Xearth,vert1,vert2,vert3,dA,ntri,A_wave,k_wave,w_wave,rho,g,Zb,EAX,dX,origin,xcg)
%EAX=Appendage eulater angle in local coordinate
%its=number of time steps to skip writing grid

x_e=Xearth(1); y_e=Xearth(2); z_e=Xearth(3);
phi=Xearth(4); theta=Xearth(5); psi=Xearth(6);
phiX=EAX(1); thetaX=EAX(2); psiX=EAX(3);


RMat=[cos(theta)*cos(psi) -cos(phi)*sin(psi)+sin(phi)*sin(theta)*cos(psi)  sin(phi)*sin(psi)+cos(phi)*sin(theta)*cos(psi); ...
      cos(theta)*sin(psi)  cos(phi)*cos(psi)+sin(phi)*sin(theta)*sin(psi) -sin(phi)*cos(psi)+cos(phi)*sin(theta)*sin(psi); ...
     -sin(theta)                             sin(phi)*cos(theta)                             cos(phi)*cos(theta)];  
RMATX=[cos(thetaX)*cos(psiX) -cos(phiX)*sin(psiX)+sin(phiX)*sin(thetaX)*cos(psiX)  sin(phiX)*sin(psiX)+cos(phiX)*sin(thetaX)*cos(psiX); ...
      cos(thetaX)*sin(psiX)  cos(phiX)*cos(psiX)+sin(phiX)*sin(thetaX)*sin(psiX) -sin(phiX)*cos(psiX)+cos(phiX)*sin(thetaX)*sin(psiX); ...
     -sin(thetaX)                             sin(phiX)*cos(thetaX)                             cos(phiX)*cos(thetaX)];  
RMATD=[cos(0)*cos(dX) -cos(0)*sin(dX)+sin(0)*sin(0)*cos(dX)  sin(0)*sin(dX)+cos(0)*sin(0)*cos(dX); ...
      cos(0)*sin(dX)  cos(0)*cos(dX)+sin(0)*sin(0)*sin(dX) -sin(0)*cos(dX)+cos(0)*sin(0)*sin(dX); ...
     -sin(0)                             sin(0)*cos(0)                             cos(0)*cos(0)];  


%Rotating the vertices to put in ship coordinate
for i=1:ntri 
    V1=[vert1(i,1); vert1(i,2); vert1(i,3);];
    V2=[vert2(i,1); vert2(i,2); vert2(i,3);];
    V3=[vert3(i,1); vert3(i,2); vert3(i,3);];
        
    %rotating to local z coordinate
    V1_o=inv(RMATX)*(V1-origin*70.2+xcg);
    V2_o=inv(RMATX)*(V2-origin*70.2+xcg);
    V3_o=inv(RMATX)*(V3-origin*70.2+xcg);
    
    %rotating for corresponding appendage deflection
    V1_x=RMATD*V1_o;
    V2_x=RMATD*V2_o;
    V3_x=RMATD*V3_o;
    
        %re-positioning the appendage to local vectors
    V1_r=RMATX*V1_x;
    V2_r=RMATX*V2_x;
    V3_r=RMATX*V3_x;
    
    %re-assigning vertices
    
    for j=1:3
    vert1(i,j)=V1_r(j)+origin(j)*70.2-xcg(j);
    vert2(i,j)=V2_r(j)+origin(j)*70.2-xcg(j);
    vert3(i,j)=V3_r(j)+origin(j)*70.2-xcg(j);
    end  
end

 
%position of mid points in earth coordinate;
mp1=zeros(ntri,3);
mp2=zeros(ntri,3);
mp3=zeros(ntri,3);
nA =zeros(ntri,3);

P1=zeros(ntri,1);
P2=zeros(ntri,1);
P3=zeros(ntri,1);

%position vector of mid points from the CG
r1=zeros(ntri,3);
r2=zeros(ntri,3);
r3=zeros(ntri,3);

v1_w=zeros(ntri,3);
v2_w=zeros(ntri,3);
v3_w=zeros(ntri,3);
n_w=zeros(ntri,3);

%Area of triangle, product of area and unit normal, position vector to each mid-point

for i=1:ntri
    %Area of each triangle
    A=[vert2(i,1)-vert1(i,1); vert2(i,2)-vert1(i,2); vert2(i,3)-vert1(i,3);];
    B=[vert3(i,1)-vert1(i,1); vert3(i,2)-vert1(i,2); vert3(i,3)-vert1(i,3);];
    n=cross(A,B)/norm(cross(A,B));
    C=[n(1); n(2); n(3);];
    %C=[normal(i,1); normal(i,2); normal(i,3);];

    
    %A*n vector calculation
    for j=1:3
        nA(i,j)=dA(i).*C(j);    
    end
    
    %position vector to each mid point of each edge
    for j=1:3
        r1(i,j)=0.5*(vert1(i,j)+vert2(i,j));
        r2(i,j)=0.5*(vert1(i,j)+vert3(i,j));
        r3(i,j)=0.5*(vert2(i,j)+vert3(i,j));
    end
end

%computing mid point location between vertices in earth coordinate
for i=1:ntri
    MP1=RMat*[r1(i,1); r1(i,2); r1(i,3);]+[x_e; y_e; z_e;];
    MP2=RMat*[r2(i,1); r2(i,2); r2(i,3);]+[x_e; y_e; z_e;];
    MP3=RMat*[r3(i,1); r3(i,2); r3(i,3);]+[x_e; y_e; z_e;];
    
    v1i=RMat*[vert1(i,1); vert1(i,2); vert1(i,3);]+[x_e; y_e; z_e;];
    v2i=RMat*[vert2(i,1); vert2(i,2); vert2(i,3);]+[x_e; y_e; z_e;];
    v3i=RMat*[vert3(i,1); vert3(i,2); vert3(i,3);]+[x_e; y_e; z_e;];
    
    for j=1:3
        v1_w(i,j)=v1i(j); v2_w(i,j)=v2i(j); v3_w(i,j)=v3i(j);
        mp1(i,j)=MP1(j);  mp2(i,j)=MP2(j);  mp3(i,j)=MP3(j);
    end
end

for i=1:ntri
    A=[v2_w(i,1)-v1_w(i,1); v2_w(i,2)-v1_w(i,2); v2_w(i,3)-v1_w(i,3);];
    B=[v3_w(i,1)-v1_w(i,1); v3_w(i,2)-v1_w(i,2); v3_w(i,3)-v1_w(i,3);];
    n=cross(A,B)/norm(cross(A,B));
    dA(i,1)=0.5*norm(cross(A,B));
    n_w(i,1)=n(1); n_w(i,2)=n(2); n_w(i,3)=n(3);
end



%computing forces and moments for each triangle
Fx_total=0; Fy_total=0; Fz_total=0;
Mx_total=0; My_total=0; Mz_total=0;

for i=1:ntri
    p1=-rho*g*(mp1(i,3)-A_wave*exp(k_wave.*mp1(i,3)).*sin(k_wave*mp1(i,1)-w_wave.*time));
    p2=-rho*g*(mp2(i,3)-A_wave*exp(k_wave.*mp2(i,3)).*sin(k_wave*mp2(i,1)-w_wave.*time));
    p3=-rho*g*(mp3(i,3)-A_wave*exp(k_wave.*mp3(i,3)).*sin(k_wave*mp3(i,1)-w_wave.*time));
    
    dFx=-nA(i,1)*(p1+p2+p3)./3;
    dFy=-nA(i,2)*(p1+p2+p3)./3;
    dFz=-nA(i,3)*(p1+p2+p3)./3;
    
    dP =-p1.*[r1(i,1); r1(i,2); r1(i,3)-Zb;]...
        -p2.*[r2(i,1); r2(i,2); r2(i,3)-Zb;]...
        -p3.*[r3(i,1); r3(i,2); r3(i,3)-Zb;];
    N =[nA(i,1); nA(i,2); nA(i,3);];
    dM=cross(dP,N);
    Fx_total=Fx_total+dFx;
    Fy_total=Fy_total+dFy;
    Fz_total=Fz_total+dFz;
    Mx_total=Mx_total+dM(1)/3;
    My_total=My_total+dM(2)/3;
    Mz_total=Mz_total+dM(3)/3;
end
end
